simulink model "HEV_Simu_V1_1"  (R2018a)
settings: Solver=ode23s  StartTime=0.0  StopTime=660  FixedStep=0.001  EnableMultiTasking=on
PreLoadFcn:
  | HevSimuVccWs_V1_PreLoad
  | %プラントモデルのコールバック・プリロード関数のバス定義
  | HEVPlant_Ptbs_V1_BusInfo
  | Engine_MapMdl_Ptbs_V1_BusInfo
  | Motor_MapMdl_Ptbs_V1_BusInfo
StartFcn:
  | tic
StopFcn:
  | toc
  | disp(['実時間の' num2str(max(tout)/toc) '倍速'])
model workspace (MAT data in the model file):
  Var = 0
undefined symbols (not defined in the file or in its folder): canChannel
libraries: canmsglib x55, canlib x35, simulink x2
(part 2 of 4)

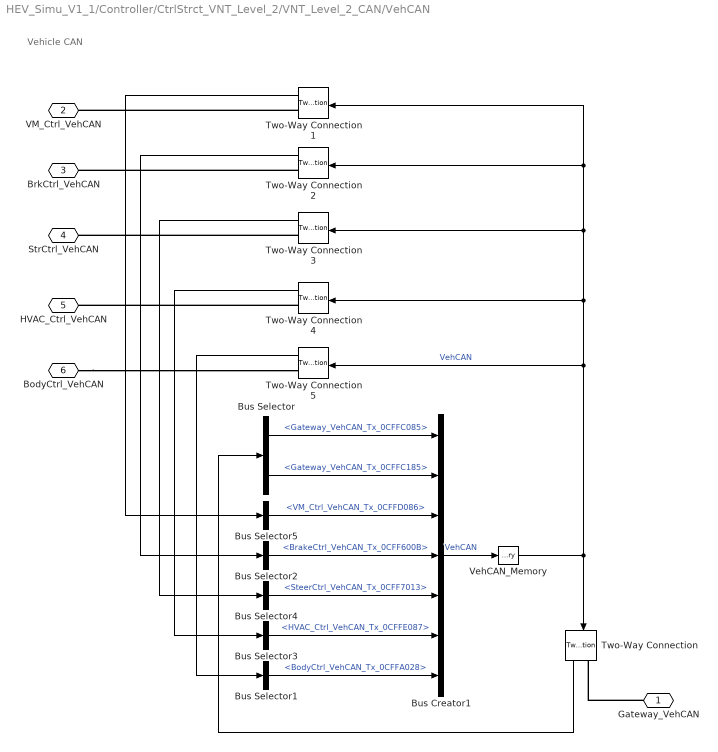
== system HEV_Simu_V1_1/Controller/CtrlStrct_VNT_Level_2/VNT_Level_2_CAN/VehCAN ==
  note: Vehicle CAN
  Bus Creator1 : BusCreator  Inputs=7
  Bus Selector : BusSelector  OutputSignals=Gateway_VehCAN_Tx_0CFFC085,Gateway_VehCAN_Tx_0CFFC185
  Bus Selector1 : BusSelector  OutputSignals=BodyCtrl_VehCAN_Tx_0CFFA028
  Bus Selector2 : BusSelector  OutputSignals=BrakeCtrl_VehCAN_Tx_0CFF600B
  Bus Selector3 : BusSelector  OutputSignals=HVAC_Ctrl_VehCAN_Tx_0CFFE087
  Bus Selector4 : BusSelector  OutputSignals=SteerCtrl_VehCAN_Tx_0CFF7013
  Bus Selector5 : BusSelector  OutputSignals=VM_Ctrl_VehCAN_Tx_0CFFD086
  Two-Way Connection{,1..5} (6 alike) : TwoWayConnection
  VehCAN_Memory : Memory
  Gateway_VehCAN : PMIOPort  Side=Right
      settings: AttributesFormatString=<Side=%<Side>>
  VM_Ctrl_VehCAN : PMIOPort  Port=2  Side=Left
      settings: AttributesFormatString=<Side=%<Side>>
  BrkCtrl_VehCAN : PMIOPort  Port=3  Side=Left
      settings: AttributesFormatString=<Side=%<Side>>
  StrCtrl_VehCAN : PMIOPort  Port=4  Side=Left
      settings: AttributesFormatString=<Side=%<Side>>
  HVAC_Ctrl_VehCAN : PMIOPort  Port=5  Side=Left
      settings: AttributesFormatString=<Side=%<Side>>
  BodyCtrl_VehCAN : PMIOPort  Port=6  Side=Left
      settings: AttributesFormatString=<Side=%<Side>>
  wires:
  Bus Creator1/1 -> VehCAN_Memory/1  "VehCAN"
  Two-Way Connection3/1 -> Bus Selector4/1
  Two-Way Connection1/1 -> Bus Selector5/1
  Two-Way Connection5/1 -> Bus Selector1/1
  VehCAN_Memory/1 -> Two-Way Connection4/1, Two-Way Connection3/1, Two-Way Connection2/1, Two-Way Connection1/1, Two-Way Connection5/1, Two-Way Connection/1  "VehCAN"
  Two-Way Connection2/1 -> Bus Selector2/1
  Two-Way Connection/1 -> Bus Selector/1
  Two-Way Connection4/1 -> Bus Selector3/1
  Bus Selector/1 -> Bus Creator1/1  "<Gateway_VehCAN_Tx_0CFFC085>"
  Bus Selector/2 -> Bus Creator1/2  "<Gateway_VehCAN_Tx_0CFFC185>"
  Bus Selector5/1 -> Bus Creator1/3  "<VM_Ctrl_VehCAN_Tx_0CFFD086>"
  Bus Selector2/1 -> Bus Creator1/4  "<BrakeCtrl_VehCAN_Tx_0CFF600B>"
  Bus Selector4/1 -> Bus Creator1/5  "<SteerCtrl_VehCAN_Tx_0CFF7013>"
  Bus Selector3/1 -> Bus Creator1/6  "<HVAC_Ctrl_VehCAN_Tx_0CFFE087>"
  Bus Selector1/1 -> Bus Creator1/7  "<BodyCtrl_VehCAN_Tx_0CFFA028>"
  connections:
  Gateway_VehCAN/RConn1 -- Two-Way Connection/RConn1
  Two-Way Connection1/RConn1 -- VM_Ctrl_VehCAN/RConn1
  Two-Way Connection2/RConn1 -- BrkCtrl_VehCAN/RConn1
  Two-Way Connection3/RConn1 -- StrCtrl_VehCAN/RConn1
  Two-Way Connection4/RConn1 -- HVAC_Ctrl_VehCAN/RConn1
  BodyCtrl_VehCAN/RConn1 -- Two-Way Connection5/RConn1

== system HEV_Simu_V1_1/Controller/CtrlStrct_VNT_Level_2/Vehicle/HEV_Control ==
  note: HEV Control
  Driver_demand : Inport
  HEV_sensor : Inport  Port=2
  HEV_Control : ModelReference  ModelNameDialog=HEV_Ctrl_V1_1.slx  SimulationMode=Normal  ModelReferenceVersion=1.0.55
  Rate Transition2 : RateTransition  Deterministic=off
      settings: AttributesFormatString=<Deterministic=%<Deterministic>>
  Rate Transition3 : RateTransition  Deterministic=off
      settings: AttributesFormatString=<Deterministic=%<Deterministic>>
  Rate Transition4 : RateTransition  Deterministic=off
      settings: AttributesFormatString=<Deterministic=%<Deterministic>>
  tag scope: HEV_Ctrl_PwtrCAN_Tx=scoped, HEV_ECU_Info=global
  wires:
  Rate Transition3/1 -> HEV_Control/1
  HEV_Control/1 -> [HEV_Ctrl_PwtrCAN_Tx]  "HEV_Ctrl_PwtrCAN_Tx"
  Rate Transition4/1 -> [HEV_ECU_Info]  "HEV_Ctrl_Info"
  HEV_Control/2 -> Rate Transition4/1
  Rate Transition2/1 -> HEV_Control/2
  HEV_sensor/1 -> Rate Transition2/1
  [HEV_Ctrl_PwtrCAN_Rx] -> HEV_Control/3
  Driver_demand/1 -> Rate Transition3/1

== system HEV_Simu_V1_1/Controller/CtrlStrct_VNT_Level_2/Vehicle/Vehicle_Motion_Control ==
  note: Vehicle Motion Control
  Env : Inport
  Rate Transition1 : RateTransition  Deterministic=off
      settings: AttributesFormatString=<Deterministic=%<Deterministic>>
  Vehicle_Motion_Control : ModelReference  ModelNameDialog=VM_Ctrl_V1_1.slx  SimulationMode=Normal  ModelReferenceVersion=0.1.26
  tag scope: VM_Ctrl_VehCAN_Tx=scoped
  wires:
  [VM_Ctrl_VehCAN_Rx] -> Vehicle_Motion_Control/2
  Env/1 -> Rate Transition1/1
  Rate Transition1/1 -> Vehicle_Motion_Control/1
  Vehicle_Motion_Control/1 -> [VM_Ctrl_VehCAN_Tx]  "VM_Ctrl_VehCAN_Tx"

== system HEV_Simu_V1_1/Controller/CtrlStrct_VNT_Level_2/Powertrain/Engine_Control/Engine_Control ==
  "DrvDem " : Inport
  "Eng_Sns " : Inport  Port=2
  EngineCtrl_PwtrCAN_Rx : Inport  Port=3
  "Info_in " : Inport  Port=4
  EngineCtrl_V1.slx : ModelReference  ModelNameDialog=EngineCtrl_V1_1.slx  SimulationMode=Normal  VariantControl=VarObj_EngEcu_Simple  ModelReferenceVersion=1.0.25
  EngineCtrl_V2.slx : ModelReference  ModelNameDialog=EngineCtrl_V2.slx  SimulationMode=Normal  VariantControl=VarObj_EngEcu_Medium  ModelReferenceVersion=1.0.8
  " EngineCtrl" : Outport
  " EngineCtrl_PwtrCAN_Tx" : Outport  Port=2
  " EngineCtrl_Info" : Outport  Port=3

== system HEV_Simu_V1_1/Controller/CtrlStrct_VNT_Level_2/Powertrain/Engine_Control/Info_in ==
  Bus Creator1 : BusCreator  Inputs=1
  Constant : Constant
  Info_in : Outport
  wires:
  Bus Creator1/1 -> Info_in/1  "Info_in"
  Constant/1 -> Bus Creator1/1  "dummy"

== system HEV_Simu_V1_1/Controller/CtrlStrct_VNT_Level_2/VNT_Level_2_CAN/Battery_Ctrl/BatteryCtrl_PwtrCAN Tx ==
  note: Function of CAN transmit
      | ・conversion fromCAN application signal to signal of CAN message
  note: Battery Control
  note: CAN transmit
  BatteryCtrl_PwtrCAN_Tx_Apli : Inport
  BatteryCtrl_PwtrCAN Pack : canmsglib/CAN Pack  CANdbFile=HEV_CANDB.dbc  MsgList=BatteryCtrl_PwtrCAN_Tx  MsgName=BatteryCtrl_PwtrCAN_Tx  MsgIDType=Extended (29-bit identifier)  MsgIdentifier=218071172  MsgLength=8  SignalInfo=BatCtrl_SOC$0$16$1$2$1$0$3.906250e-03$0$0$100$#  NSignals=1  StartBits=str2num('[int32(0)]')  SignalSizes=str2num('[int32(16)]')  ByteOrders=str2num('[int32(1)]')  DataTypes=str2num('[int32(2)]')  MultiplexTypes=str2num('[int32(1)]')  MultiplexValues=str2num('[double(0)]')  Factors=str2num('[double(3.906250e-03)]')  Offsets=str2num('[double(0)]')  Minimums=str2num('[double(0)]')  Maximums=str2num('[double(100)]')  Remote=off  ApplyMinMax=off  BusOutput=off
      settings: AttributesFormatString=<CANdbFile = %<CANdbFile>>  SourceProductName=Simulink Real-Time  SourceProductBaseCode=XP  DataFormat=CANdb specified signals
  BatteryCtrl_PwtrCAN Transmit : canlib/CAN Transmit  BlockHandle=27972.0004  DeviceMenu=MathWorks Virtual 1 (Channel 1)  Device=MathWorks Virtual 1 (Channel 1)  ObjConstructor=canChannel('MathWorks','Virtual 1',1)  EnablePeriodicTransmit=on  MessagePeriod=0.05
      settings: AttributesFormatString=<MessagePeriod = %<MessagePeriod>>  SourceProductName=Vehicle Network Toolbox  SourceProductBaseCode=VN
  Bus Creator1 : BusCreator  Inputs=1
  Bus Selector1 : BusSelector  OutputSignals=BatCtrl_SOC
  BatteryCtrl_PwtrCAN_Tx : Outport
  wires:
  BatteryCtrl_PwtrCAN Pack/1 -> BatteryCtrl_PwtrCAN Transmit/1, Bus Creator1/1  "BatteryCtrl_PwtrCAN_Tx_0CFF8084"
  Bus Creator1/1 -> BatteryCtrl_PwtrCAN_Tx/1  "BatteryCtrl_PwtrCAN_Tx"
  Bus Selector1/1 -> BatteryCtrl_PwtrCAN Pack/1  "<BatCtrl_SOC>"
  BatteryCtrl_PwtrCAN_Tx_Apli/1 -> Bus Selector1/1

== system HEV_Simu_V1_1/Controller/CtrlStrct_VNT_Level_2/VNT_Level_2_CAN/Battery_Ctrl/BatteryCtrl_PwtrCAN_Rx ==
  note: Function of CAN receive
      | ・CAN message selection
      | ・conversion from CAN signal to CAN application signal with bus object
  note: Battery Control
  note: CAN receive
  PwtrCAN : Inport
  BatteryCtrl_PwtrCAN Receive : canlib/CAN Receive  BlockHandle=27987.0004  DeviceMenu=MathWorks Virtual 1 (Channel 1)  Device=MathWorks Virtual 1 (Channel 1)  ObjConstructor=canChannel('MathWorks','Virtual 1',1)  EnableStandardIDsFilter=off  StandardIDs=0  EnableExtendedIDsFilter=off  ExtendedIDs=0  SampleTime=0.05  MsgsPerTimestep=all  StdIDsCombo=Allow all  ExtIDsCombo=Allow all  InternalFilterUpdateStatus=on  BusOutput=off
      settings: AttributesFormatString=<SampleTime = %<SampleTime>>  SourceProductName=Vehicle Network Toolbox  SourceProductBaseCode=VN
  BatteryCtrl_PwtrCAN_Receive_50ms : Subsystem
  Bus Creator5 : BusCreator  Inputs=1
  Bus Selector2 : BusSelector  OutputSignals=HEV_Ctrl_PwtrCAN_Tx_0CFF2082
  Rate Transition1 : RateTransition  Deterministic=off
      settings: AttributesFormatString=<Deterministic=%<Deterministic>>
  Terminator : Terminator
  BatteryCtrl_PwtrCAN_Rx : Outport
  wires:
  Bus Creator5/1 -> Rate Transition1/1
  Rate Transition1/1 -> BatteryCtrl_PwtrCAN_Rx/1  "BatteryCtrl_PwtrCAN_Rx"
  PwtrCAN/1 -> Bus Selector2/1
  Bus Selector2/1 -> Terminator/1  "<HEV_Ctrl_PwtrCAN_Tx_0CFF2082>"
  BatteryCtrl_PwtrCAN_Receive_50ms/1(HEVCtrl_Motor_torque_request) -> Bus Creator5/1
  BatteryCtrl_PwtrCAN Receive/1 -> BatteryCtrl_PwtrCAN_Receive_50ms/Trigger
  BatteryCtrl_PwtrCAN Receive/2 -> BatteryCtrl_PwtrCAN_Receive_50ms/1(PwtrCAN_Msg)

== system HEV_Simu_V1_1/Controller/CtrlStrct_VNT_Level_2/VNT_Level_2_CAN/Body_Ctrl/BodyCtrl_VehCAN Tx ==
  note: Function of CAN transmit
      | ・conversion fromCAN application signal to signal of CAN message
  note: CAN transmit
  note: Body Control
  BodyCtrl_VehCAN_Tx_Apli : Inport
  BodyCtrl_VehCAN Pack : canmsglib/CAN Pack  CANdbFile=HEV_CANDB.dbc  MsgList=BodyCtrl_VehCAN_Tx  MsgName=BodyCtrl_VehCAN_Tx  MsgIDType=Extended (29-bit identifier)  MsgIdentifier=218079272  MsgLength=8  SignalInfo=BdyCtrl_Door_open_flag$1$1$1$2$1$0$1$0$0$1$#BdyCtrl_Engine_hood_open_flag$1$1$1$2$1$0$1$0$0$1$#BdyCtrl_Idlestop_cancel$0$1$1$2$1$0$1$0$0$1$#  NSignals=3  StartBits=str2num('[int32(1);int32(1);int32(0)]')  SignalSizes=str2num('[int32(1);int32(1);int32(1)]')  ByteOrders=str2num('[int32(1);int32(1);int32(1)]')  DataTypes=str2num('[int32(2);int32(2);int32(2)]')  MultiplexTypes=str2num('[int32(1);int32(1);int32(1)]')  MultiplexValues=str2num('[double(0);double(0);double(0)]')  Factors=str2num('[double(1);double(1);double(1)]')  Offsets=str2num('[double(0);double(0);double(0)]')  Minimums=str2num('[double(0);double(0);double(0)]')  Maximums=str2num('[double(1);double(1);double(1)]')  Remote=off  ApplyMinMax=off  BusOutput=off
      settings: AttributesFormatString=<CANdbFile = %<CANdbFile>>  SourceProductName=Simulink Real-Time  SourceProductBaseCode=XP  DataFormat=CANdb specified signals
  BodyCtrl_VehCAN Transmit : canlib/CAN Transmit  BlockHandle=28033.0004  DeviceMenu=MathWorks Virtual 1 (Channel 1)  Device=MathWorks Virtual 1 (Channel 1)  ObjConstructor=canChannel('MathWorks','Virtual 1',1)  EnablePeriodicTransmit=on  MessagePeriod=0.05
      settings: AttributesFormatString=<MessagePeriod = %<MessagePeriod>>  SourceProductName=Vehicle Network Toolbox  SourceProductBaseCode=VN
  Bus Creator1 : BusCreator  Inputs=1
  Bus Selector2 : BusSelector  OutputSignals=BdyCtrl_Idlestop_cancel,BdyCtrl_Engine_hood_open_flag,BdyCtrl_Door_open_flag
  BodyCtrl_VehCAN_Tx : Outport
  wires:
  Bus Selector2/1 -> BodyCtrl_VehCAN Pack/1  "<BdyCtrl_Idlestop_cancel>"
  Bus Selector2/2 -> BodyCtrl_VehCAN Pack/2  "<BdyCtrl_Engine_hood_open_flag>"
  Bus Creator1/1 -> BodyCtrl_VehCAN_Tx/1  "BodyCtrl_VehCAN_Tx"
  Bus Selector2/3 -> BodyCtrl_VehCAN Pack/3  "<BdyCtrl_Door_open_flag>"
  BodyCtrl_VehCAN Pack/1 -> BodyCtrl_VehCAN Transmit/1, Bus Creator1/1  "BodyCtrl_VehCAN_Tx_0CFFA028"
  BodyCtrl_VehCAN_Tx_Apli/1 -> Bus Selector2/1

== system HEV_Simu_V1_1/Controller/CtrlStrct_VNT_Level_2/VNT_Level_2_CAN/Body_Ctrl/BodyCtrl_VehCAN_Rx ==
  note: CAN receive
  note: Body Control
  note: Function of CAN receive
      | ・CAN message selection
      | ・conversion from CAN signal to CAN application signal with bus object
  VehCAN : Inport
  BodyCtrl_VehCAN Receive : canlib/CAN Receive  BlockHandle=28050.0004  DeviceMenu=MathWorks Virtual 1 (Channel 1)  Device=MathWorks Virtual 1 (Channel 1)  ObjConstructor=canChannel('MathWorks','Virtual 1',1)  EnableStandardIDsFilter=off  StandardIDs=0  EnableExtendedIDsFilter=off  ExtendedIDs=0  SampleTime=0.05  MsgsPerTimestep=all  StdIDsCombo=Allow all  ExtIDsCombo=Allow all  InternalFilterUpdateStatus=on  BusOutput=off
      settings: AttributesFormatString=<SampleTime = %<SampleTime>>  SourceProductName=Vehicle Network Toolbox  SourceProductBaseCode=VN
  BodyCtrl_VehCAN_Receive_50ms : Subsystem
  Bus Creator : BusCreator  Inputs=3
  Bus Selector4 : BusSelector  OutputSignals=Gateway_VehCAN_Tx_0CFFC185
  Bus Selector7 : BusSelector  OutputSignals=BrakeCtrl_VehCAN_Tx_0CFF600B
  Rate Transition1 : RateTransition  Deterministic=off
      settings: AttributesFormatString=<Deterministic=%<Deterministic>>
  Terminator : Terminator
  Terminator1 : Terminator
  BodyCtrl_VehCAN_Rx : Outport
  wires:
  VehCAN/1 -> Bus Selector4/1, Bus Selector7/1
  Bus Creator/1 -> Rate Transition1/1
  Rate Transition1/1 -> BodyCtrl_VehCAN_Rx/1  "BodyCtrl_VehCAN_Rx"
  Bus Selector7/1 -> Terminator/1  "<BrakeCtrl_VehCAN_Tx_0CFF600B>"
  Bus Selector4/1 -> Terminator1/1  "<Gateway_VehCAN_Tx_0CFFC185>"
  BodyCtrl_VehCAN_Receive_50ms/1(BrkCtrl_Vehicle_speed) -> Bus Creator/1
  BodyCtrl_VehCAN_Receive_50ms/2(EngCtrl_Engine_speed) -> Bus Creator/2
  BodyCtrl_VehCAN_Receive_50ms/3(HEVCtrl_IdleStop_status) -> Bus Creator/3
  BodyCtrl_VehCAN Receive/1 -> BodyCtrl_VehCAN_Receive_50ms/Trigger
  BodyCtrl_VehCAN Receive/2 -> BodyCtrl_VehCAN_Receive_50ms/1(VehCAN_Msg)

== system HEV_Simu_V1_1/Controller/CtrlStrct_VNT_Level_2/VNT_Level_2_CAN/Brake_Ctrl/BrakeCtrl_VehCAN Tx ==
  note: CAN transmit
  note: Brake Control
  note: Function of CAN transmit
      | ・conversion fromCAN application signal to signal of CAN message
  BrakeCtrl_VehCAN_Tx_Apli : Inport
  BrakeCtrl_VehCAN Pack : canmsglib/CAN Pack  CANdbFile=HEV_CANDB.dbc  MsgList=BrakeCtrl_VehCAN_Tx  MsgName=BrakeCtrl_VehCAN_Tx  MsgIDType=Extended (29-bit identifier)  MsgIdentifier=218062859  MsgLength=8  SignalInfo=BrkCtrl_Regen_brake_torque_reque$16$16$1$1$1$0$1.000000e-02$0$-300$300$#BrkCtrl_Vehicle_speed$0$16$1$2$1$0$1.000000e-01$0$0$180$#  NSignals=2  StartBits=str2num('[int32(16);int32(0)]')  SignalSizes=str2num('[int32(16);int32(16)]')  ByteOrders=str2num('[int32(1);int32(1)]')  DataTypes=str2num('[int32(1);int32(2)]')  MultiplexTypes=str2num('[int32(1);int32(1)]')  MultiplexValues=str2num('[double(0);double(0)]')  Factors=str2num('[double(1.000000e-02);double(1.000000e-01)]')  Offsets=str2num('[double(0);double(0)]')  Minimums=str2num('[double(-300);double(0)]')  Maximums=str2num('[double(300);double(180)]')  Remote=off  ApplyMinMax=off  BusOutput=off
      settings: AttributesFormatString=<CANdbFile = %<CANdbFile>>  SourceProductName=Simulink Real-Time  SourceProductBaseCode=XP  DataFormat=CANdb specified signals
  BrakeCtrl_VehCAN Transmit : canlib/CAN Transmit  BlockHandle=28275.0004  DeviceMenu=MathWorks Virtual 1 (Channel 1)  Device=MathWorks Virtual 1 (Channel 1)  ObjConstructor=canChannel('MathWorks','Virtual 1',1)  EnablePeriodicTransmit=on  MessagePeriod=0.01
      settings: AttributesFormatString=<MessagePeriod = %<MessagePeriod>>  SourceProductName=Vehicle Network Toolbox  SourceProductBaseCode=VN
  Bus Creator1 : BusCreator  Inputs=1
  Bus Selector4 : BusSelector  OutputSignals=BrkCtrl_Regen_brake_torque_request,BrkCtrl_Vehicle_speed
  BrakeCtrl_VehCAN_Tx : Outport
  wires:
  Bus Selector4/2 -> BrakeCtrl_VehCAN Pack/2  "<BrkCtrl_Vehicle_speed>"
  BrakeCtrl_VehCAN_Tx_Apli/1 -> Bus Selector4/1
  Bus Creator1/1 -> BrakeCtrl_VehCAN_Tx/1  "BrakeCtrl_VehCAN_Tx"
  Bus Selector4/1 -> BrakeCtrl_VehCAN Pack/1  "<BrkCtrl_Regen_brake_torque_request>"
  BrakeCtrl_VehCAN Pack/1 -> BrakeCtrl_VehCAN Transmit/1, Bus Creator1/1  "BrakeCtrl_VehCAN_Tx_0CFF600B"

== system HEV_Simu_V1_1/Controller/CtrlStrct_VNT_Level_2/VNT_Level_2_CAN/Brake_Ctrl/BrakeCtrl_VehCAN_Rx ==
  note: CAN receive
  note: Brake Control
  note: Function of CAN receive
      | ・CAN message selection
      | ・conversion from CAN signal to CAN application signal with bus object
  VehCAN : Inport
  BrakeCtrl_VehCAN Receive : canlib/CAN Receive  BlockHandle=28304.0004  DeviceMenu=MathWorks Virtual 1 (Channel 1)  Device=MathWorks Virtual 1 (Channel 1)  ObjConstructor=canChannel('MathWorks','Virtual 1',1)  EnableStandardIDsFilter=off  StandardIDs=0  EnableExtendedIDsFilter=off  ExtendedIDs=0  SampleTime=0.01  MsgsPerTimestep=all  StdIDsCombo=Allow all  ExtIDsCombo=Allow all  InternalFilterUpdateStatus=on  BusOutput=off
      settings: AttributesFormatString=<SampleTime = %<SampleTime>>  SourceProductName=Vehicle Network Toolbox  SourceProductBaseCode=VN
  BrakeCtrl_VehCAN_Receive_10ms : Subsystem
  Bus Creator : BusCreator  Inputs=4
  Bus Selector2 : BusSelector  OutputSignals=VM_Ctrl_VehCAN_Tx_0CFFD086
  Bus Selector3 : BusSelector  OutputSignals=Gateway_VehCAN_Tx_0CFFC085
  Rate Transition1 : RateTransition  Deterministic=off
      settings: AttributesFormatString=<Deterministic=%<Deterministic>>
  Terminator : Terminator
  Terminator1 : Terminator
  BrakeCtrl_VehCAN_Rx : Outport
  wires:
  VehCAN/1 -> Bus Selector2/1, Bus Selector3/1
  Bus Creator/1 -> Rate Transition1/1
  Rate Transition1/1 -> BrakeCtrl_VehCAN_Rx/1  "BrakeCtrl_VehCAN_Rx"
  Bus Selector3/1 -> Terminator/1  "<Gateway_VehCAN_Tx_0CFFC085>"
  Bus Selector2/1 -> Terminator1/1  "<VM_Ctrl_VehCAN_Tx_0CFFD086>"
  BrakeCtrl_VehCAN_Receive_10ms/1(HEVCtrl_Regen_brake_torque_available) -> Bus Creator/1
  BrakeCtrl_VehCAN_Receive_10ms/2(HEVCtrl_Regen_brake_torque_actual) -> Bus Creator/2
  BrakeCtrl_VehCAN_Receive_10ms/3(VMCtrl_BrakeForceStatus) -> Bus Creator/3
  BrakeCtrl_VehCAN_Receive_10ms/4(VMCtrl_BrakeForceCmnd) -> Bus Creator/4
  BrakeCtrl_VehCAN Receive/1 -> BrakeCtrl_VehCAN_Receive_10ms/Trigger
  BrakeCtrl_VehCAN Receive/2 -> BrakeCtrl_VehCAN_Receive_10ms/1(VehCAN_Msg)

== system HEV_Simu_V1_1/Controller/CtrlStrct_VNT_Level_2/VNT_Level_2_CAN/Engine_Ctrl/EngineCtrl_PwtrCAN Tx ==
  note: Function of CAN transmit
      | ・conversion fromCAN application signal to signal of CAN message
  note: Engine Control
  note: CAN transmit
  EngineCtrl_PwtrCAN_Tx_Apli : Inport
  Bus Creator1 : BusCreator  Inputs=1
  Bus Selector3 : BusSelector  OutputSignals=EngCtrl_Engine_speed,EngCtrl_Engine_torque_actual
  EngineCtrl_PwtrCAN Pack : canmsglib/CAN Pack  CANdbFile=HEV_CANDB.dbc  MsgList=EngineCtrl_PwtrCAN_Tx  MsgName=EngineCtrl_PwtrCAN_Tx  MsgIDType=Extended (29-bit identifier)  MsgIdentifier=218050560  MsgLength=8  SignalInfo=EngCtrl_Engine_speed$0$16$1$2$1$0$1.250000e-01$0$0$8192$#EngCtrl_Engine_torque_actual$16$16$1$1$1$0$1.562500e-02$0$-300$300$#  NSignals=2  StartBits=str2num('[int32(0);int32(16)]')  SignalSizes=str2num('[int32(16);int32(16)]')  ByteOrders=str2num('[int32(1);int32(1)]')  DataTypes=str2num('[int32(2);int32(1)]')  MultiplexTypes=str2num('[int32(1);int32(1)]')  MultiplexValues=str2num('[double(0);double(0)]')  Factors=str2num('[double(1.250000e-01);double(1.562500e-02)]')  Offsets=str2num('[double(0);double(0)]')  Minimums=str2num('[double(0);double(-300)]')  Maximums=str2num('[double(8192);double(300)]')  Remote=off  ApplyMinMax=off  BusOutput=off
      settings: AttributesFormatString=<CANdbFile = %<CANdbFile>>  SourceProductName=Simulink Real-Time  SourceProductBaseCode=XP  DataFormat=CANdb specified signals
  EngineCtrl_PwtrCAN Transmit : canlib/CAN Transmit  BlockHandle=28379.0004  DeviceMenu=MathWorks Virtual 1 (Channel 1)  Device=MathWorks Virtual 1 (Channel 1)  ObjConstructor=canChannel('MathWorks','Virtual 1',1)  EnablePeriodicTransmit=on  MessagePeriod=0.01
      settings: AttributesFormatString=<MessagePeriod = %<MessagePeriod>>  SourceProductName=Vehicle Network Toolbox  SourceProductBaseCode=VN
  EngineCtrl_PwtrCAN_Tx : Outport
  wires:
  EngineCtrl_PwtrCAN Pack/1 -> Bus Creator1/1  "EngineCtrl_PwtrCAN_Tx_0CFF3000"
  Bus Selector3/2 -> EngineCtrl_PwtrCAN Pack/2  "<EngCtrl_Engine_torque_actual>"
  Bus Selector3/1 -> EngineCtrl_PwtrCAN Pack/1  "<EngCtrl_Engine_speed>"
  EngineCtrl_PwtrCAN_Tx_Apli/1 -> Bus Selector3/1
  Bus Creator1/1 -> EngineCtrl_PwtrCAN Transmit/1, EngineCtrl_PwtrCAN_Tx/1  "EngineCtrl_PwtrCAN_Tx"

== system HEV_Simu_V1_1/Controller/CtrlStrct_VNT_Level_2/VNT_Level_2_CAN/Engine_Ctrl/EngineCtrl_PwtrCAN_Rx ==
  note: Function of CAN receive
      | ・CAN message selection
      | ・conversion from CAN signal to CAN application signal with bus object
  note: Engine Control
  note: CAN receive
  PwtrCAN : Inport
  Bus Creator5 : BusCreator  Inputs=4
  EngineCtrl_PwtrCAN Receive : canlib/CAN Receive  BlockHandle=28394.0004  DeviceMenu=MathWorks Virtual 1 (Channel 1)  Device=MathWorks Virtual 1 (Channel 1)  ObjConstructor=canChannel('MathWorks','Virtual 1',1)  EnableStandardIDsFilter=off  StandardIDs=0  EnableExtendedIDsFilter=off  ExtendedIDs=0  SampleTime=0.01  MsgsPerTimestep=all  StdIDsCombo=Allow all  ExtIDsCombo=Allow all  InternalFilterUpdateStatus=on  BusOutput=off
      settings: AttributesFormatString=<SampleTime = %<SampleTime>>  SourceProductName=Vehicle Network Toolbox  SourceProductBaseCode=VN
  EngineCtrl_PwtrCAN_Receive_10ms : Subsystem
  Rate Transition1 : RateTransition  Deterministic=off
      settings: AttributesFormatString=<Deterministic=%<Deterministic>>
  Terminator : Terminator
  EngineCtrl_PwtrCAN_Rx : Outport
  wires:
  Bus Creator5/1 -> Rate Transition1/1
  Rate Transition1/1 -> EngineCtrl_PwtrCAN_Rx/1  "EngineCtrl_PwtrCAN_Rx"
  PwtrCAN/1 -> Terminator/1
  EngineCtrl_PwtrCAN_Receive_10ms/1(HEVCtrl_Engine_torque_request) -> Bus Creator5/1
  EngineCtrl_PwtrCAN_Receive_10ms/2(HEVCtrl_IdleStop_preparation_request) -> Bus Creator5/2
  EngineCtrl_PwtrCAN_Receive_10ms/3(HEVCtrl_IdleStop_request) -> Bus Creator5/3
  EngineCtrl_PwtrCAN_Receive_10ms/4(HEVCtrl_IdleStop_status) -> Bus Creator5/4
  EngineCtrl_PwtrCAN Receive/1 -> EngineCtrl_PwtrCAN_Receive_10ms/Trigger
  EngineCtrl_PwtrCAN Receive/2 -> EngineCtrl_PwtrCAN_Receive_10ms/1(PwtrCAN_Msg)

== system HEV_Simu_V1_1/Controller/CtrlStrct_VNT_Level_2/VNT_Level_2_CAN/Gateway/Gateway InfoCAN ==
  note: Gateway Info CAN
  VehCAN : Inport
  VehSpd : Inport  Port=2
  Bus Creator : BusCreator  Inputs=1
  Bus Selector8 : BusSelector  OutputSignals=BrakeCtrl_VehCAN_Tx_0CFF600B
  Gatewary_InfoCAN Transmit : canlib/CAN Transmit  BlockHandle=28493.0004  DeviceMenu=MathWorks Virtual 1 (Channel 1)  Device=MathWorks Virtual 1 (Channel 1)  ObjConstructor=canChannel('MathWorks','Virtual 1',1)  EnablePeriodicTransmit=on  MessagePeriod=0.1
      settings: AttributesFormatString=<MessagePeriod = %<MessagePeriod>>  SourceProductName=Vehicle Network Toolbox  SourceProductBaseCode=VN
  Gateway_InfoCAN Pack : canmsglib/CAN Pack  CANdbFile=HEV_CANDB.dbc  MsgList=Gateway_InfoCAN_Tx  MsgName=Gateway_InfoCAN_Tx  MsgIDType=Extended (29-bit identifier)  MsgIdentifier=218099848  MsgLength=8  SignalInfo=BrkCtrl_Vehicle_speed_G1$0$16$1$2$1$0$1.000000e-01$0$0$180$#  NSignals=1  StartBits=str2num('[int32(0)]')  SignalSizes=str2num('[int32(16)]')  ByteOrders=str2num('[int32(1)]')  DataTypes=str2num('[int32(2)]')  MultiplexTypes=str2num('[int32(1)]')  MultiplexValues=str2num('[double(0)]')  Factors=str2num('[double(1.000000e-01)]')  Offsets=str2num('[double(0)]')  Minimums=str2num('[double(0)]')  Maximums=str2num('[double(180)]')  Remote=off  ApplyMinMax=off  BusOutput=off
      settings: AttributesFormatString=<CANdbFile = %<CANdbFile>>  SourceProductName=Simulink Real-Time  SourceProductBaseCode=XP  DataFormat=CANdb specified signals
  Gateway_VehCAN Unpack : canmsglib/CAN Unpack  CANdbFile=HEV_CANDB.dbc  MsgList=BrakeCtrl_VehCAN_Tx  MsgName=BrakeCtrl_VehCAN_Tx  MsgIDType=Extended (29-bit identifier)  MsgIdentifier=218062859  MsgLength=8  SignalInfo=BrkCtrl_Regen_brake_torque_reque$16$16$1$1$1$0$1.000000e-02$0$-300$300$#BrkCtrl_Vehicle_speed$0$16$1$2$1$0$1.000000e-01$0$0$180$#  NSignals=2  IDPort=off  TimestampPort=off  ErrorPort=off  RemotePort=off  LengthPort=off  StatusPort=off  StartBits=str2num('[int32(16);int32(0)]')  SignalSizes=str2num('[int32(16);int32(16)]')  ByteOrders=str2num('[int32(1);int32(1)]')  DataTypes=str2num('[int32(1);int32(2)]')  MultiplexTypes=str2num('[int32(1);int32(1)]')  MultiplexValues=str2num('[double(0);double(0)]')  Factors=str2num('[double(1.000000e-02);double(1.000000e-01)]')  Offsets=str2num('[double(0);double(0)]')  Minimums=str2num('[double(-300);double(0)]')  Maximums=str2num('[double(300);double(180)]')  ApplyMinMax=off
      settings: AttributesFormatString=<CANdbFile = %<CANdbFile>>  SourceProductName=Simulink Real-Time  SourceProductBaseCode=XP  DataFormat=CANdb specified signals
  Terminator1 : Terminator
  Terminator4 : Terminator
  Gateway_InfoCAN : Outport
  wires:
  VehCAN/1 -> Bus Selector8/1
  Bus Creator/1 -> Gateway_InfoCAN/1  "Gateway_InfoCAN"
  Bus Selector8/1 -> Gateway_VehCAN Unpack/1  "<BrakeCtrl_VehCAN_Tx_0CFF600B>"
  Gateway_VehCAN Unpack/1 -> Terminator4/1  "BrkCtrl_Regen_brake_torque_request"
  Gateway_VehCAN Unpack/2 -> Terminator1/1  "BrkCtrl_Vehicle_speed"
  VehSpd/1 -> Gateway_InfoCAN Pack/1
  Gateway_InfoCAN Pack/1 -> Bus Creator/1, Gatewary_InfoCAN Transmit/1  "Gateway_InfoCAN_Tx_0CFFC485"

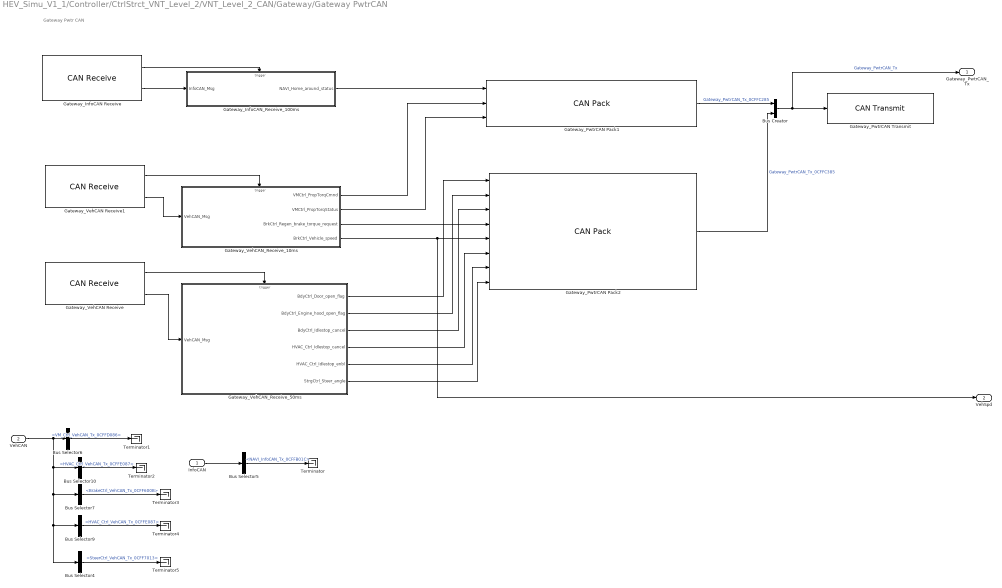
== system HEV_Simu_V1_1/Controller/CtrlStrct_VNT_Level_2/VNT_Level_2_CAN/Gateway/Gateway PwtrCAN ==
  note: Gateway Pwtr CAN
  InfoCAN : Inport
  VehCAN : Inport  Port=2
  Bus Creator : BusCreator  Inputs=2
  Bus Selector10 : BusSelector  OutputSignals=HVAC_Ctrl_VehCAN_Tx_0CFFE087
  Bus Selector4 : BusSelector  OutputSignals=SteerCtrl_VehCAN_Tx_0CFF7013
  Bus Selector5 : BusSelector  OutputSignals=NAVI_InfoCAN_Tx_0CFFB01C
  Bus Selector6 : BusSelector  OutputSignals=VM_Ctrl_VehCAN_Tx_0CFFD086
  Bus Selector7 : BusSelector  OutputSignals=BrakeCtrl_VehCAN_Tx_0CFF600B
  Bus Selector9 : BusSelector  OutputSignals=HVAC_Ctrl_VehCAN_Tx_0CFFE087
  Gateway_InfoCAN Receive : canlib/CAN Receive  BlockHandle=28547.0004  DeviceMenu=MathWorks Virtual 1 (Channel 1)  Device=MathWorks Virtual 1 (Channel 1)  ObjConstructor=canChannel('MathWorks','Virtual 1',1)  EnableStandardIDsFilter=off  StandardIDs=0  EnableExtendedIDsFilter=off  ExtendedIDs=0  SampleTime=0.1  MsgsPerTimestep=all  StdIDsCombo=Allow all  ExtIDsCombo=Allow all  InternalFilterUpdateStatus=on  BusOutput=off
      settings: AttributesFormatString=<SampleTime = %<SampleTime>>  SourceProductName=Vehicle Network Toolbox  SourceProductBaseCode=VN
  Gateway_InfoCAN_Receive_100ms : Subsystem
  Gateway_PwtrCAN Pack1 : canmsglib/CAN Pack  CANdbFile=HEV_CANDB.dbc  MsgList=Gateway_PwtrCAN_Tx_1  MsgName=Gateway_PwtrCAN_Tx_1  MsgIDType=Extended (29-bit identifier)  MsgIdentifier=218088069  MsgLength=8  SignalInfo=NAVI_Home_around_status_G$0$16$1$2$1$0$1$0$0$65535$#VMCtrl_PropTorqCmnd_G$24$16$1$1$1$0$1.000000e-02$0$-300$300$#VMCtrl_PropTorqStatus_G$16$8$1$2$1$0$1$0$0$7$#  NSignals=3  StartBits=str2num('[int32(0);int32(24);int32(16)]')  SignalSizes=str2num('[int32(16);int32(16);int32(8)]')  ByteOrders=str2num('[int32(1);int32(1);int32(1)]')  DataTypes=str2num('[int32(2);int32(1);int32(2)]')  MultiplexTypes=str2num('[int32(1);int32(1);int32(1)]')  MultiplexValues=str2num('[double(0);double(0);double(0)]')  Factors=str2num('[double(1);double(1.000000e-02);double(1)]')  Offsets=str2num('[double(0);double(0);double(0)]')  Minimums=str2num('[double(0);double(-300);double(0)]')  Maximums=str2num('[double(65535);double(300);double(7)]')  Remote=off  ApplyMinMax=off  BusOutput=off
      settings: AttributesFormatString=<CANdbFile = %<CANdbFile>>  SourceProductName=Simulink Real-Time  SourceProductBaseCode=XP  DataFormat=CANdb specified signals
  Gateway_PwtrCAN Pack2 : canmsglib/CAN Pack  CANdbFile=HEV_CANDB.dbc  MsgList=Gateway_PwtrCAN_Tx_2  MsgName=Gateway_PwtrCAN_Tx_2  MsgIDType=Extended (29-bit identifier)  MsgIdentifier=218088325  MsgLength=8  SignalInfo=BdyCtrl_Door_open_flag_G$60$1$1$2$1$0$1$0$0$1$#BdyCtrl_Engine_hood_open_flg_G$59$1$1$2$1$0$1$0$0$1$#BdyCtrl_Idlestop_cancel_G$58$1$1$2$1$0$1$0$0$1$#BrkCtrl_Regen_brake_torque_re_G$16$16$1$1$1$0$1.000000e-02$0$-300$300$#BrkCtrl_Vehicle_speed_G$0$16$1$2$1$0$1.000000e-01$0$0$180$#HVAC_Ctrl_Idlestop_cancel_G$57$1$1$2$1$0$1$0$0$1$#HVAC_Ctrl_Idlestop_enbl_G$56$1$1$2$1$0$1$0$0$1$#StrgCtrl_Steer_angle_G$32$16$1$1$1$0$3.125000e-02$0$-720$720$#  NSignals=8  StartBits=str2num('[int32(60);int32(59);int32(58);int32(16);int32(0);int32(57);int32(56);int32(32)]')  SignalSizes=str2num('[int32(1);int32(1);int32(1);int32(16);int32(16);int32(1);int32(1);int32(16)]')  ByteOrders=str2num('[int32(1);int32(1);int32(1);int32(1);int32(1);int32(1);int32(1);int32(1)]')  DataTypes=str2num('[int32(2);int32(2);int32(2);int32(1);int32(2);int32(2);int32(2);int32(1)]')  MultiplexTypes=str2num('[int32(1);int32(1);int32(1);int32(1);int32(1);int32(1);int32(1);int32(1)]')  MultiplexValues=str2num('[double(0);double(0);double(0);double(0);double(0);double(0);double(0);double(0)]')  Factors=str2num('[double(1);double(1);double(1);double(1.000000e-02);double(1.000000e-01);double(1);double(1);double(3.125000e-02)]')  Offsets=str2num('[double(0);double(0);double(0);double(0);double(0);double(0);double(0);double(0)]')  Minimums=str2num('[double(0);double(0);double(0);double(-300);double(0);double(0);double(0);double(-720)]')  Maximums=str2num('[double(1);double(1);double(1);double(300);double(180);double(1);double(1);double(720)]')  Remote=off  ApplyMinMax=off  BusOutput=off
      settings: AttributesFormatString=<CANdbFile = %<CANdbFile>>  SourceProductName=Simulink Real-Time  SourceProductBaseCode=XP  DataFormat=CANdb specified signals
  Gateway_PwtrCAN Transmit : canlib/CAN Transmit  BlockHandle=28561.0004  DeviceMenu=MathWorks Virtual 1 (Channel 1)  Device=MathWorks Virtual 1 (Channel 1)  ObjConstructor=canChannel('MathWorks','Virtual 1',1)  EnablePeriodicTransmit=on  MessagePeriod=0.01
      settings: AttributesFormatString=<MessagePeriod = %<MessagePeriod>>  SourceProductName=Vehicle Network Toolbox  SourceProductBaseCode=VN
  Gateway_VehCAN Receive : canlib/CAN Receive  BlockHandle=28562.0004  DeviceMenu=MathWorks Virtual 1 (Channel 1)  Device=MathWorks Virtual 1 (Channel 1)  ObjConstructor=canChannel('MathWorks','Virtual 1',1)  EnableStandardIDsFilter=off  StandardIDs=0  EnableExtendedIDsFilter=off  ExtendedIDs=0  SampleTime=0.05  MsgsPerTimestep=all  StdIDsCombo=Allow all  ExtIDsCombo=Allow all  InternalFilterUpdateStatus=on  BusOutput=off
      settings: AttributesFormatString=<SampleTime = %<SampleTime>>  SourceProductName=Vehicle Network Toolbox  SourceProductBaseCode=VN
  Gateway_VehCAN Receive1 : canlib/CAN Receive  BlockHandle=28563.0004  DeviceMenu=MathWorks Virtual 1 (Channel 1)  Device=MathWorks Virtual 1 (Channel 1)  ObjConstructor=canChannel('MathWorks','Virtual 1',1)  EnableStandardIDsFilter=off  StandardIDs=0  EnableExtendedIDsFilter=off  ExtendedIDs=0  SampleTime=0.01  MsgsPerTimestep=all  StdIDsCombo=Allow all  ExtIDsCombo=Allow all  InternalFilterUpdateStatus=on  BusOutput=off
      settings: AttributesFormatString=<SampleTime = %<SampleTime>>  SourceProductName=Vehicle Network Toolbox  SourceProductBaseCode=VN
  Gateway_VehCAN_Receive_10ms : Subsystem
  Gateway_VehCAN_Receive_50ms : Subsystem
  Terminator{,1..5} (6 alike) : Terminator
  Gateway_PwtrCAN_Tx : Outport
  VehSpd : Outport  Port=2
  wires:
  InfoCAN/1 -> Bus Selector5/1
  Bus Selector5/1 -> Terminator/1  "<NAVI_InfoCAN_Tx_0CFFB01C>"
  Gateway_InfoCAN_Receive_100ms/1(NAVI_Home_around_status) -> Gateway_PwtrCAN Pack1/1
  Gateway_InfoCAN Receive/2 -> Gateway_InfoCAN_Receive_100ms/1(InfoCAN_Msg)
  Gateway_InfoCAN Receive/1 -> Gateway_InfoCAN_Receive_100ms/Trigger
  VehCAN/1 -> Bus Selector10/1, Bus Selector7/1, Bus Selector4/1, Bus Selector9/1, Bus Selector6/1
  Bus Selector4/1 -> Terminator5/1  "<SteerCtrl_VehCAN_Tx_0CFF7013>"
  Bus Selector9/1 -> Terminator4/1  "<HVAC_Ctrl_VehCAN_Tx_0CFFE087>"
  Bus Selector7/1 -> Terminator3/1  "<BrakeCtrl_VehCAN_Tx_0CFF600B>"
  Bus Selector6/1 -> Terminator1/1  "<VM_Ctrl_VehCAN_Tx_0CFFD086>"
  Gateway_VehCAN Receive1/2 -> Gateway_VehCAN_Receive_10ms/1(VehCAN_Msg)
  Gateway_VehCAN_Receive_10ms/2(VMCtrl_PropTorqStatus) -> Gateway_PwtrCAN Pack1/3
  Gateway_VehCAN_Receive_10ms/1(VMCtrl_PropTorqCmnd) -> Gateway_PwtrCAN Pack1/2
  Gateway_VehCAN_Receive_10ms/4(BrkCtrl_Vehicle_speed) -> VehSpd/1, Gateway_PwtrCAN Pack2/5
  Gateway_VehCAN_Receive_10ms/3(BrkCtrl_Regen_brake_torque_request) -> Gateway_PwtrCAN Pack2/4
  Gateway_VehCAN Receive1/1 -> Gateway_VehCAN_Receive_10ms/Trigger
  Bus Selector10/1 -> Terminator2/1  "<HVAC_Ctrl_VehCAN_Tx_0CFFE087>"
  Gateway_VehCAN_Receive_50ms/6(StrgCtrl_Steer_angle) -> Gateway_PwtrCAN Pack2/8
  Gateway_VehCAN_Receive_50ms/5(HVAC_Ctrl_Idlestop_enbl) -> Gateway_PwtrCAN Pack2/7
  Gateway_VehCAN_Receive_50ms/4(HVAC_Ctrl_Idlestop_cancel) -> Gateway_PwtrCAN Pack2/6
  Gateway_VehCAN_Receive_50ms/3(BdyCtrl_Idlestop_cancel) -> Gateway_PwtrCAN Pack2/3
  Gateway_VehCAN_Receive_50ms/2(BdyCtrl_Engine_hood_open_flag) -> Gateway_PwtrCAN Pack2/2
  Gateway_VehCAN_Receive_50ms/1(BdyCtrl_Door_open_flag) -> Gateway_PwtrCAN Pack2/1
  Gateway_VehCAN Receive/2 -> Gateway_VehCAN_Receive_50ms/1(VehCAN_Msg)
  Gateway_VehCAN Receive/1 -> Gateway_VehCAN_Receive_50ms/Trigger
  Gateway_PwtrCAN Pack2/1 -> Bus Creator/2  "Gateway_PwtrCAN_Tx_0CFFC385"
  Gateway_PwtrCAN Pack1/1 -> Bus Creator/1  "Gateway_PwtrCAN_Tx_0CFFC285"
  Bus Creator/1 -> Gateway_PwtrCAN Transmit/1, Gateway_PwtrCAN_Tx/1  "Gateway_PwtrCAN_Tx"

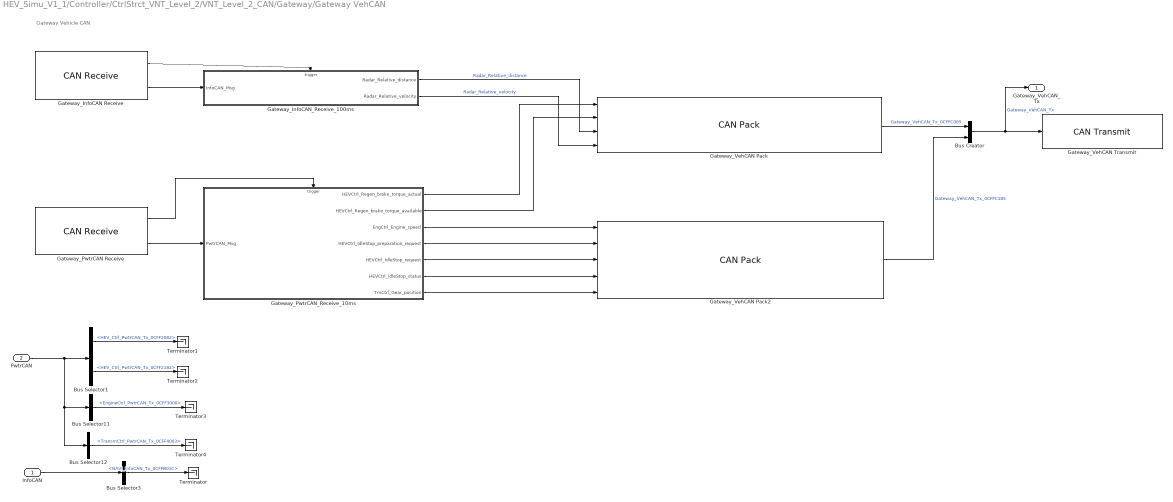
== system HEV_Simu_V1_1/Controller/CtrlStrct_VNT_Level_2/VNT_Level_2_CAN/Gateway/Gateway VehCAN ==
  note: Gateway Vehicle CAN
  InfoCAN : Inport
  PwtrCAN : Inport  Port=2
  Bus Creator : BusCreator  Inputs=2
  Bus Selector1 : BusSelector  OutputSignals=HEV_Ctrl_PwtrCAN_Tx_0CFF2082,HEV_Ctrl_PwtrCAN_Tx_0CFF2182
  Bus Selector11 : BusSelector  OutputSignals=EngineCtrl_PwtrCAN_Tx_0CFF3000
  Bus Selector12 : BusSelector  OutputSignals=TransmCtrl_PwtrCAN_Tx_0CFF4003
  Bus Selector3 : BusSelector  OutputSignals=NAVI_InfoCAN_Tx_0CFFB01C
  Gateway_InfoCAN Receive : canlib/CAN Receive  BlockHandle=28672.0004  DeviceMenu=MathWorks Virtual 1 (Channel 1)  Device=MathWorks Virtual 1 (Channel 1)  ObjConstructor=canChannel('MathWorks','Virtual 1',1)  EnableStandardIDsFilter=off  StandardIDs=0  EnableExtendedIDsFilter=off  ExtendedIDs=0  SampleTime=0.1  MsgsPerTimestep=all  StdIDsCombo=Allow all  ExtIDsCombo=Allow all  InternalFilterUpdateStatus=on  BusOutput=off
      settings: AttributesFormatString=<SampleTime = %<SampleTime>>  SourceProductName=Vehicle Network Toolbox  SourceProductBaseCode=VN
  Gateway_InfoCAN_Receive_100ms : Subsystem
  Gateway_PwtrCAN Receive : canlib/CAN Receive  BlockHandle=28682.0004  DeviceMenu=MathWorks Virtual 1 (Channel 1)  Device=MathWorks Virtual 1 (Channel 1)  ObjConstructor=canChannel('MathWorks','Virtual 1',1)  EnableStandardIDsFilter=off  StandardIDs=0  EnableExtendedIDsFilter=off  ExtendedIDs=0  SampleTime=0.01  MsgsPerTimestep=all  StdIDsCombo=Allow all  ExtIDsCombo=Allow all  InternalFilterUpdateStatus=on  BusOutput=off
      settings: AttributesFormatString=<SampleTime = %<SampleTime>>  SourceProductName=Vehicle Network Toolbox  SourceProductBaseCode=VN
  Gateway_PwtrCAN_Receive_10ms : Subsystem
  Gateway_VehCAN Pack : canmsglib/CAN Pack  CANdbFile=HEV_CANDB.dbc  MsgList=Gateway_VehCAN_Tx_1  MsgName=Gateway_VehCAN_Tx_1  MsgIDType=Extended (29-bit identifier)  MsgIdentifier=218087557  MsgLength=8  SignalInfo=HEVCtrl_Regen_brake_torque_act_G$48$16$1$1$1$0$6.250000e-02$0$-300$3000$#HEVCtrl_Regen_brake_torque_ave_G$32$16$1$1$1$0$6.250000e-02$0$-300$3000$#Radar_Relative_distance_G$0$16$1$2$1$0$1.000000e-02$0$0$500$#Radar_Relative_velocity_G$16$16$1$1$1$0$1.000000e-02$0$-50$50$#  NSignals=4  StartBits=str2num('[int32(48);int32(32);int32(0);int32(16)]')  SignalSizes=str2num('[int32(16);int32(16);int32(16);int32(16)]')  ByteOrders=str2num('[int32(1);int32(1);int32(1);int32(1)]')  DataTypes=str2num('[int32(1);int32(1);int32(2);int32(1)]')  MultiplexTypes=str2num('[int32(1);int32(1);int32(1);int32(1)]')  MultiplexValues=str2num('[double(0);double(0);double(0);double(0)]')  Factors=str2num('[double(6.250000e-02);double(6.250000e-02);double(1.000000e-02);double(1.000000e-02)]')  Offsets=str2num('[double(0);double(0);double(0);double(0)]')  Minimums=str2num('[double(-300);double(-300);double(0);double(-50)]')  Maximums=str2num('[double(3000);double(3000);double(500);double(50)]')  Remote=off  ApplyMinMax=off  BusOutput=off
      settings: AttributesFormatString=<CANdbFile = %<CANdbFile>>  SourceProductName=Simulink Real-Time  SourceProductBaseCode=XP  DataFormat=CANdb specified signals
  Gateway_VehCAN Pack2 : canmsglib/CAN Pack  CANdbFile=HEV_CANDB.dbc  MsgList=Gateway_VehCAN_Tx_2  MsgName=Gateway_VehCAN_Tx_2  MsgIDType=Extended (29-bit identifier)  MsgIdentifier=218087813  MsgLength=8  SignalInfo=EngCtrl_Engine_speed_G$0$16$1$2$1$0$1.250000e-01$0$0$8192$#HEV_IdleStopCtrl_preparation_r_G$24$1$1$2$1$0$1$0$0$1$#HEV_IdleStopCtrl_request_G$25$1$1$2$1$0$1$0$0$1$#HEV_IdleStopCtrl_status_G$26$1$1$2$1$0$1$0$0$1$#TmCtrl_Gear_position_G$16$8$1$2$1$0$1$0$0$5$#  NSignals=5  StartBits=str2num('[int32(0);int32(24);int32(25);int32(26);int32(16)]')  SignalSizes=str2num('[int32(16);int32(1);int32(1);int32(1);int32(8)]')  ByteOrders=str2num('[int32(1);int32(1);int32(1);int32(1);int32(1)]')  DataTypes=str2num('[int32(2);int32(2);int32(2);int32(2);int32(2)]')  MultiplexTypes=str2num('[int32(1);int32(1);int32(1);int32(1);int32(1)]')  MultiplexValues=str2num('[double(0);double(0);double(0);double(0);double(0)]')  Factors=str2num('[double(1.250000e-01);double(1);double(1);double(1);double(1)]')  Offsets=str2num('[double(0);double(0);double(0);double(0);double(0)]')  Minimums=str2num('[double(0);double(0);double(0);double(0);double(0)]')  Maximums=str2num('[double(8192);double(1);double(1);double(1);double(5)]')  Remote=off  ApplyMinMax=off  BusOutput=off
      settings: AttributesFormatString=<CANdbFile = %<CANdbFile>>  SourceProductName=Simulink Real-Time  SourceProductBaseCode=XP  DataFormat=CANdb specified signals
  Gateway_VehCAN Transmit : canlib/CAN Transmit  BlockHandle=28721.0004  DeviceMenu=MathWorks Virtual 1 (Channel 1)  Device=MathWorks Virtual 1 (Channel 1)  ObjConstructor=canChannel('MathWorks','Virtual 1',1)  EnablePeriodicTransmit=on  MessagePeriod=0.05
      settings: AttributesFormatString=<MessagePeriod = %<MessagePeriod>>  SourceProductName=Vehicle Network Toolbox  SourceProductBaseCode=VN
  Terminator{,1..4} (5 alike) : Terminator
  Gateway_VehCAN_Tx : Outport
  wires:
  InfoCAN/1 -> Bus Selector3/1
  Bus Selector3/1 -> Terminator/1  "<NAVI_InfoCAN_Tx_0CFFB01C>"
  Gateway_InfoCAN Receive/2 -> Gateway_InfoCAN_Receive_100ms/1(InfoCAN_Msg)
  Gateway_InfoCAN Receive/1 -> Gateway_InfoCAN_Receive_100ms/Trigger
  Gateway_InfoCAN_Receive_100ms/2(Radar_Relative_velocity) -> Gateway_VehCAN Pack/4  "Radar_Relative_velocity"
  Gateway_InfoCAN_Receive_100ms/1(Radar_Relative_distance) -> Gateway_VehCAN Pack/3  "Radar_Relative_distance"
  Bus Creator/1 -> Gateway_VehCAN Transmit/1, Gateway_VehCAN_Tx/1  "Gateway_VehCAN_Tx"
  Gateway_VehCAN Pack2/1 -> Bus Creator/2  "Gateway_VehCAN_Tx_0CFFC185"
  Gateway_VehCAN Pack/1 -> Bus Creator/1  "Gateway_VehCAN_Tx_0CFFC085"
  PwtrCAN/1 -> Bus Selector11/1, Bus Selector12/1, Bus Selector1/1
  Bus Selector1/1 -> Terminator1/1  "<HEV_Ctrl_PwtrCAN_Tx_0CFF2082>"
  Bus Selector1/2 -> Terminator2/1  "<HEV_Ctrl_PwtrCAN_Tx_0CFF2182>"
  Bus Selector11/1 -> Terminator3/1  "<EngineCtrl_PwtrCAN_Tx_0CFF3000>"
  Bus Selector12/1 -> Terminator4/1  "<TransmCtrl_PwtrCAN_Tx_0CFF4003>"
  Gateway_PwtrCAN_Receive_10ms/1(HEVCtrl_Regen_brake_torque_actual) -> Gateway_VehCAN Pack/1
  Gateway_PwtrCAN_Receive_10ms/2(HEVCtrl_Regen_brake_torque_available) -> Gateway_VehCAN Pack/2
  Gateway_PwtrCAN_Receive_10ms/3(EngCtrl_Engine_speed) -> Gateway_VehCAN Pack2/1
  Gateway_PwtrCAN_Receive_10ms/4(HEVCtrl_IdleStop_preparation_request) -> Gateway_VehCAN Pack2/2
  Gateway_PwtrCAN_Receive_10ms/5(HEVCtrl_IdleStop_request) -> Gateway_VehCAN Pack2/3
  Gateway_PwtrCAN_Receive_10ms/6(HEVCtrl_IdleStop_status) -> Gateway_VehCAN Pack2/4
  Gateway_PwtrCAN_Receive_10ms/7(TmCtrl_Gear_position) -> Gateway_VehCAN Pack2/5
  Gateway_PwtrCAN Receive/1 -> Gateway_PwtrCAN_Receive_10ms/Trigger
  Gateway_PwtrCAN Receive/2 -> Gateway_PwtrCAN_Receive_10ms/1(PwtrCAN_Msg)

== system HEV_Simu_V1_1/Controller/CtrlStrct_VNT_Level_2/VNT_Level_2_CAN/Gateway/Info Hub ==
  note: Info Hub
  InfoCAN : Inport
  VehCAN : Inport  Port=2
  PwtrCAN : Inport  Port=3
  Bus Creator3 : BusCreator  Inputs=3
  tag scope: CAN=scoped
  wires:
  PwtrCAN/1 -> Bus Creator3/3
  Bus Creator3/1 -> [CAN]
  VehCAN/1 -> Bus Creator3/2
  InfoCAN/1 -> Bus Creator3/1

== system HEV_Simu_V1_1/Controller/CtrlStrct_VNT_Level_2/VNT_Level_2_CAN/HEV_Ctrl/HEV_Ctrl_PwtrCAN Tx ==
  note: Function of CAN transmit
      | ・conversion fromCAN application signal to signal of CAN message
  note: HEV control
  note: CAN transmit
  HEV_Ctrl_PwtrCAN_Tx_Apli : Inport
  Bus Creator : BusCreator  Inputs=2
  Bus Selector1 : BusSelector  OutputSignals=HEVCtrl_Engine_torque_request,HEVCtrl_Motor_torque_request,HEVCtrl_Regen_brake_torque_actual,HEVCtrl_Regen_brake_torque_available,HEVCtrl_IdleStop_preparation_request,HEVCtrl_IdleStop_request,HEVCtrl_IdleStop_status
  HEV_Ctrl_PwtrCAN Pack : canmsglib/CAN Pack  CANdbFile=HEV_CANDB.dbc  MsgList=HEV_Ctrl_PwtrCAN_Tx_1  MsgName=HEV_Ctrl_PwtrCAN_Tx_1  MsgIDType=Extended (29-bit identifier)  MsgIdentifier=218046594  MsgLength=8  SignalInfo=HEVCtrl_Engine_torque_request$0$16$1$1$1$0$1.562500e-02$0$-300$300$#HEVCtrl_Motor_torque_request$16$16$1$1$1$0$1.562500e-02$0$-300$300$#HEVCtrl_Regen_brake_torque_actua$48$16$1$1$1$0$6.250000e-02$0$-300$3000$#HEVCtrl_Regen_brake_torque_avail$32$16$1$1$1$0$6.250000e-02$0$-300$3000$#  NSignals=4  StartBits=str2num('[int32(0);int32(16);int32(48);int32(32)]')  SignalSizes=str2num('[int32(16);int32(16);int32(16);int32(16)]')  ByteOrders=str2num('[int32(1);int32(1);int32(1);int32(1)]')  DataTypes=str2num('[int32(1);int32(1);int32(1);int32(1)]')  MultiplexTypes=str2num('[int32(1);int32(1);int32(1);int32(1)]')  MultiplexValues=str2num('[double(0);double(0);double(0);double(0)]')  Factors=str2num('[double(1.562500e-02);double(1.562500e-02);double(6.250000e-02);double(6.250000e-02)]')  Offsets=str2num('[double(0);double(0);double(0);double(0)]')  Minimums=str2num('[double(-300);double(-300);double(-300);double(-300)]')  Maximums=str2num('[double(300);double(300);double(3000);double(3000)]')  Remote=off  ApplyMinMax=off  BusOutput=off
      settings: AttributesFormatString=<CANdbFile = %<CANdbFile>>  SourceProductName=Simulink Real-Time  SourceProductBaseCode=XP  DataFormat=CANdb specified signals
  HEV_Ctrl_PwtrCAN Pack2 : canmsglib/CAN Pack  CANdbFile=HEV_CANDB.dbc  MsgList=HEV_Ctrl_PwtrCAN_Tx_2  MsgName=HEV_Ctrl_PwtrCAN_Tx_2  MsgIDType=Extended (29-bit identifier)  MsgIdentifier=218046850  MsgLength=8  SignalInfo=HEV_IdleStopCtrl_preparation_req$0$1$1$2$1$0$1$0$0$1$#HEV_IdleStopCtrl_request$1$1$1$2$1$0$1$0$0$1$#HEV_IdleStopCtrl_status$2$1$1$2$1$0$1$0$0$1$#  NSignals=3  StartBits=str2num('[int32(0);int32(1);int32(2)]')  SignalSizes=str2num('[int32(1);int32(1);int32(1)]')  ByteOrders=str2num('[int32(1);int32(1);int32(1)]')  DataTypes=str2num('[int32(2);int32(2);int32(2)]')  MultiplexTypes=str2num('[int32(1);int32(1);int32(1)]')  MultiplexValues=str2num('[double(0);double(0);double(0)]')  Factors=str2num('[double(1);double(1);double(1)]')  Offsets=str2num('[double(0);double(0);double(0)]')  Minimums=str2num('[double(0);double(0);double(0)]')  Maximums=str2num('[double(1);double(1);double(1)]')  Remote=off  ApplyMinMax=off  BusOutput=off
      settings: AttributesFormatString=<CANdbFile = %<CANdbFile>>  SourceProductName=Simulink Real-Time  SourceProductBaseCode=XP  DataFormat=CANdb specified signals
  HEV_Ctrl_PwtrCAN Transmit : canlib/CAN Transmit  BlockHandle=28827.0004  DeviceMenu=MathWorks Virtual 1 (Channel 1)  Device=MathWorks Virtual 1 (Channel 1)  ObjConstructor=canChannel('MathWorks','Virtual 1',1)  EnablePeriodicTransmit=on  MessagePeriod=0.01
      settings: AttributesFormatString=<MessagePeriod = %<MessagePeriod>>  SourceProductName=Vehicle Network Toolbox  SourceProductBaseCode=VN
  HEV_Ctrl_PwtrCAN_Tx : Outport
  wires:
  Bus Selector1/2 -> HEV_Ctrl_PwtrCAN Pack/2  "<HEVCtrl_Motor_torque_request>"
  Bus Selector1/1 -> HEV_Ctrl_PwtrCAN Pack/1  "<HEVCtrl_Engine_torque_request>"
  Bus Selector1/3 -> HEV_Ctrl_PwtrCAN Pack/3  "<HEVCtrl_Regen_brake_torque_actual>"
  Bus Selector1/6 -> HEV_Ctrl_PwtrCAN Pack2/2  "<HEVCtrl_IdleStop_request>"
  Bus Selector1/4 -> HEV_Ctrl_PwtrCAN Pack/4  "<HEVCtrl_Regen_brake_torque_available>"
  Bus Selector1/5 -> HEV_Ctrl_PwtrCAN Pack2/1  "<HEVCtrl_IdleStop_preparation_request>"
  HEV_Ctrl_PwtrCAN Pack2/1 -> Bus Creator/2  "HEV_Ctrl_PwtrCAN_Tx_0CFF2182"
  HEV_Ctrl_PwtrCAN Pack/1 -> Bus Creator/1  "HEV_Ctrl_PwtrCAN_Tx_0CFF2082"
  Bus Selector1/7 -> HEV_Ctrl_PwtrCAN Pack2/3  "<HEVCtrl_IdleStop_status>"
  Bus Creator/1 -> HEV_Ctrl_PwtrCAN Transmit/1, HEV_Ctrl_PwtrCAN_Tx/1  "HEV_Ctrl_PwtrCAN_Tx"
  HEV_Ctrl_PwtrCAN_Tx_Apli/1 -> Bus Selector1/1

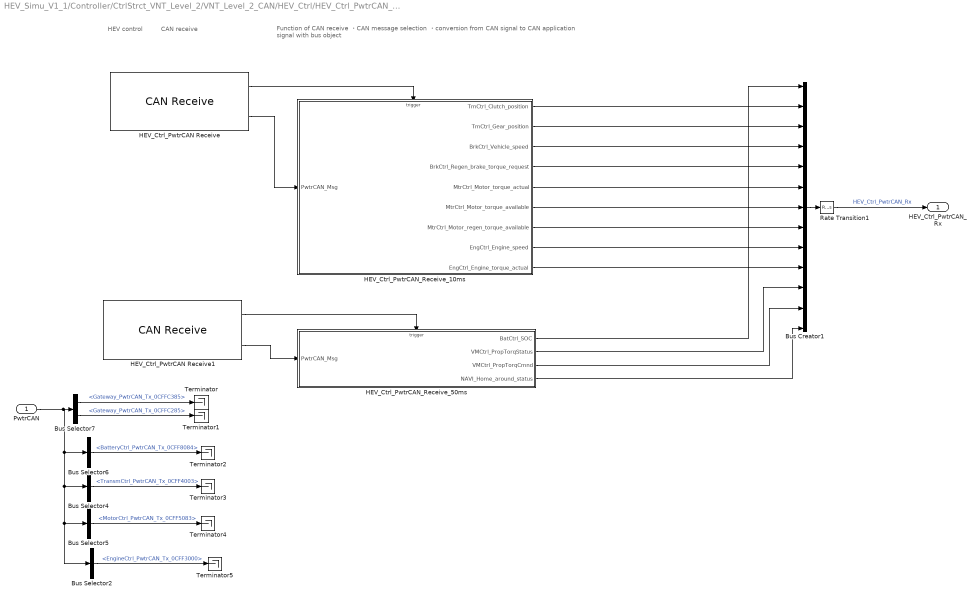
== system HEV_Simu_V1_1/Controller/CtrlStrct_VNT_Level_2/VNT_Level_2_CAN/HEV_Ctrl/HEV_Ctrl_PwtrCAN_Rx ==
  note: Function of CAN receive
      | ・CAN message selection
      | ・conversion from CAN signal to CAN application signal with bus object
  note: HEV control
  note: CAN receive
  PwtrCAN : Inport
  Bus Creator1 : BusCreator  Inputs=13  OutDataTypeStr=Bus: HEV_Ctrl_PwtrCAN_Rx_Bus
  Bus Selector2 : BusSelector  OutputSignals=EngineCtrl_PwtrCAN_Tx_0CFF3000
  Bus Selector4 : BusSelector  OutputSignals=TransmCtrl_PwtrCAN_Tx_0CFF4003
  Bus Selector5 : BusSelector  OutputSignals=MotorCtrl_PwtrCAN_Tx_0CFF5083
  Bus Selector6 : BusSelector  OutputSignals=BatteryCtrl_PwtrCAN_Tx_0CFF8084
  Bus Selector7 : BusSelector  OutputSignals=Gateway_PwtrCAN_Tx_0CFFC385,Gateway_PwtrCAN_Tx_0CFFC285
  HEV_Ctrl_PwtrCAN Receive : canlib/CAN Receive  BlockHandle=28853.0004  DeviceMenu=MathWorks Virtual 1 (Channel 1)  Device=MathWorks Virtual 1 (Channel 1)  ObjConstructor=canChannel('MathWorks','Virtual 1',1)  EnableStandardIDsFilter=off  StandardIDs=0  EnableExtendedIDsFilter=off  ExtendedIDs=0  SampleTime=0.01  MsgsPerTimestep=all  StdIDsCombo=Allow all  ExtIDsCombo=Allow all  InternalFilterUpdateStatus=on  BusOutput=off
      settings: AttributesFormatString=<SampleTime = %<SampleTime>>  SourceProductName=Vehicle Network Toolbox  SourceProductBaseCode=VN
  HEV_Ctrl_PwtrCAN Receive1 : canlib/CAN Receive  BlockHandle=28854.0004  DeviceMenu=MathWorks Virtual 1 (Channel 1)  Device=MathWorks Virtual 1 (Channel 1)  ObjConstructor=canChannel('MathWorks','Virtual 1',1)  EnableStandardIDsFilter=off  StandardIDs=0  EnableExtendedIDsFilter=off  ExtendedIDs=0  SampleTime=0.05  MsgsPerTimestep=all  StdIDsCombo=Allow all  ExtIDsCombo=Allow all  InternalFilterUpdateStatus=on  BusOutput=off
      settings: AttributesFormatString=<SampleTime = %<SampleTime>>  SourceProductName=Vehicle Network Toolbox  SourceProductBaseCode=VN
  HEV_Ctrl_PwtrCAN_Receive_10ms : Subsystem
  HEV_Ctrl_PwtrCAN_Receive_50ms : Subsystem
  Rate Transition1 : RateTransition  Deterministic=off
      settings: AttributesFormatString=<Deterministic=%<Deterministic>>
  Terminator{,1..5} (6 alike) : Terminator
  HEV_Ctrl_PwtrCAN_Rx : Outport
  wires:
  PwtrCAN/1 -> Bus Selector2/1, Bus Selector5/1, Bus Selector4/1, Bus Selector6/1, Bus Selector7/1
  Bus Creator1/1 -> Rate Transition1/1
  Rate Transition1/1 -> HEV_Ctrl_PwtrCAN_Rx/1  "HEV_Ctrl_PwtrCAN_Rx"
  Bus Selector7/2 -> Terminator1/1  "<Gateway_PwtrCAN_Tx_0CFFC285>"
  Bus Selector6/1 -> Terminator2/1  "<BatteryCtrl_PwtrCAN_Tx_0CFF8084>"
  HEV_Ctrl_PwtrCAN_Receive_50ms/1(BatCtrl_SOC) -> Bus Creator1/1
  HEV_Ctrl_PwtrCAN_Receive_50ms/2(VMCtrl_PropTorqStatus) -> Bus Creator1/11
  HEV_Ctrl_PwtrCAN_Receive_50ms/3(VMCtrl_PropTorqCmnd) -> Bus Creator1/12
  HEV_Ctrl_PwtrCAN_Receive_50ms/4(NAVI_Home_around_status) -> Bus Creator1/13
  Bus Selector7/1 -> Terminator/1  "<Gateway_PwtrCAN_Tx_0CFFC385>"
  Bus Selector4/1 -> Terminator3/1  "<TransmCtrl_PwtrCAN_Tx_0CFF4003>"
  Bus Selector5/1 -> Terminator4/1  "<MotorCtrl_PwtrCAN_Tx_0CFF5083>"
  Bus Selector2/1 -> Terminator5/1  "<EngineCtrl_PwtrCAN_Tx_0CFF3000>"
  HEV_Ctrl_PwtrCAN_Receive_10ms/1(TmCtrl_Clutch_position) -> Bus Creator1/2
  HEV_Ctrl_PwtrCAN_Receive_10ms/2(TmCtrl_Gear_position) -> Bus Creator1/3
  HEV_Ctrl_PwtrCAN_Receive_10ms/3(BrkCtrl_Vehicle_speed) -> Bus Creator1/4
  HEV_Ctrl_PwtrCAN_Receive_10ms/4(BrkCtrl_Regen_brake_torque_request) -> Bus Creator1/5
  HEV_Ctrl_PwtrCAN_Receive_10ms/5(MtrCtrl_Motor_torque_actual) -> Bus Creator1/6
  HEV_Ctrl_PwtrCAN_Receive_10ms/6(MtrCtrl_Motor_torque_available) -> Bus Creator1/7
  HEV_Ctrl_PwtrCAN_Receive_10ms/7(MtrCtrl_Motor_regen_torque_available) -> Bus Creator1/8
  HEV_Ctrl_PwtrCAN_Receive_10ms/8(EngCtrl_Engine_speed) -> Bus Creator1/9
  HEV_Ctrl_PwtrCAN_Receive_10ms/9(EngCtrl_Engine_torque_actual) -> Bus Creator1/10
  HEV_Ctrl_PwtrCAN Receive/1 -> HEV_Ctrl_PwtrCAN_Receive_10ms/Trigger
  HEV_Ctrl_PwtrCAN Receive1/1 -> HEV_Ctrl_PwtrCAN_Receive_50ms/Trigger
  HEV_Ctrl_PwtrCAN Receive1/2 -> HEV_Ctrl_PwtrCAN_Receive_50ms/1(PwtrCAN_Msg)
  HEV_Ctrl_PwtrCAN Receive/2 -> HEV_Ctrl_PwtrCAN_Receive_10ms/1(PwtrCAN_Msg)
